simulink library "spacecraft_simulink_library"  (Simulink 7.8)
settings: Solver=ode45  SolverMode=SingleTasking  StartTime=0.0  StopTime=10.0  RelTol=1e-3
undefined symbols (not defined in the file or in its folder): I_sc, Krcs, q_bi0, sun_sensor_model_type, Trcs_saturation, w_bi0
settings Model: Creator=HARDAC_S  LastModifiedBy=HARDAC_S

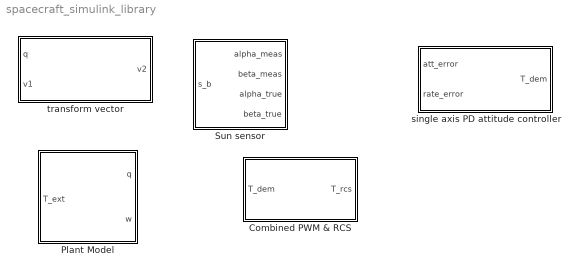
== system spacecraft_simulink_library ==
  Combined PWM & RCS : Subsystem  mask{T_deadband=[0 0 0], T_saturation=Trcs_saturation, K_rcs=[Krcs Krcs Krcs]}
      mask prompts: T_deadband "Torque deadbands [X Y Z] [Nm]"; T_saturation "Torque saturation [X Y Z] [Nm]"; K_rcs "RCS gain [X Y Z]"
  Plant Model : Subsystem
  Sun sensor : Subsystem
  single axis PD attitude controller : Subsystem  mask{Kp=0, Kd=0}
      mask prompts: Kp "Proportional gain Kp"; Kd "Derivative gain Kd"
  transform vector : MATLAB Function  TreatAsAtomicUnit=on

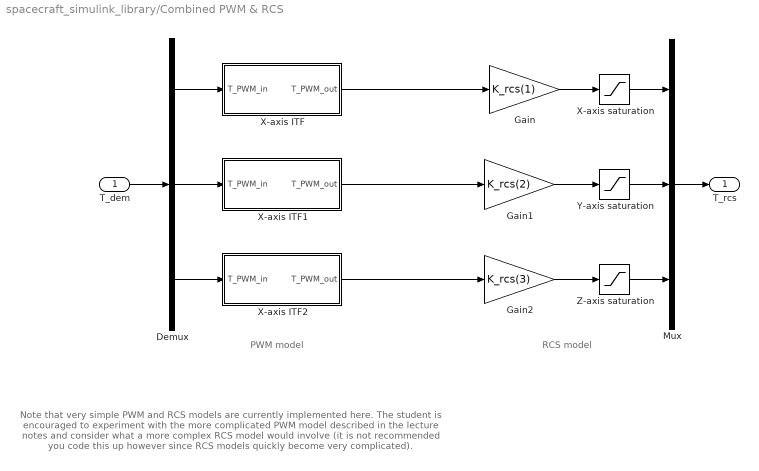
== system spacecraft_simulink_library/Combined PWM & RCS ==
  note: Note that very simple PWM and RCS models are currently implemented here. The student is
      | encouraged to experiment with the more complicated PWM model described in the lecture
      | notes and consider what a more complex RCS model would involve (it is not recommended
      | you code this up however since RCS models quickly become very complicated).
  note: RCS model
  note: PWM model
  T_dem : Inport
  Demux : Demux  Outputs=3
  Gain : Gain  Gain=K_rcs(1)  SaturateOnIntegerOverflow=on  OutDataTypeStr=Inherit: Same as input  ParamDataTypeStr=Inherit: Same as input
  Gain1 : Gain  Gain=K_rcs(2)  SaturateOnIntegerOverflow=on  OutDataTypeStr=Inherit: Same as input  ParamDataTypeStr=Inherit: Same as input
  Gain2 : Gain  Gain=K_rcs(3)  SaturateOnIntegerOverflow=on  OutDataTypeStr=Inherit: Same as input  ParamDataTypeStr=Inherit: Same as input
  Mux : Mux  Inputs=3
  X-axis ITF : Subsystem  mask{T_db=T_deadband(1)}
      mask prompts: T_db "Torque deadband [Nm]"
  X-axis ITF1 : Subsystem  mask{T_db=T_deadband(2)}
      mask prompts: T_db "Torque deadband [Nm]"
  X-axis ITF2 : Subsystem  mask{T_db=T_deadband(3)}
      mask prompts: T_db "Torque deadband [Nm]"
  X-axis saturation : Saturate  UpperLimit=+T_saturation(1)  LowerLimit=-T_saturation(1)
  Y-axis saturation : Saturate  UpperLimit=T_saturation(2)  LowerLimit=-T_saturation(2)
  Z-axis saturation : Saturate  UpperLimit=T_saturation(3)  LowerLimit=-T_saturation(3)
  T_rcs : Outport
  wires:
  Gain2/1 -> Z-axis saturation/1
  Gain1/1 -> Y-axis saturation/1
  Gain/1 -> X-axis saturation/1
  X-axis ITF2/1(T_PWM_out) -> Gain2/1
  X-axis ITF1/1(T_PWM_out) -> Gain1/1
  X-axis ITF/1(T_PWM_out) -> Gain/1
  T_dem/1 -> Demux/1
  Demux/3 -> X-axis ITF2/1(T_PWM_in)
  Demux/2 -> X-axis ITF1/1(T_PWM_in)
  Demux/1 -> X-axis ITF/1(T_PWM_in)
  Z-axis saturation/1 -> Mux/3
  Y-axis saturation/1 -> Mux/2
  X-axis saturation/1 -> Mux/1
  Mux/1 -> T_rcs/1

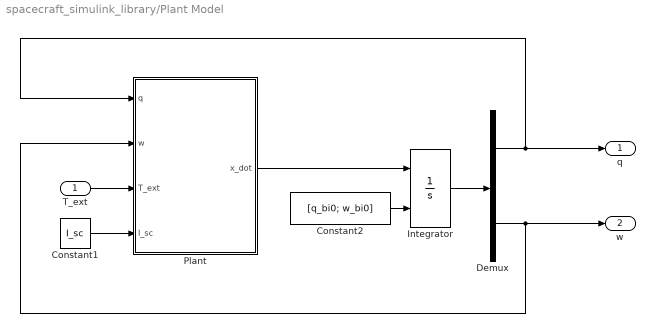
== system spacecraft_simulink_library/Plant Model ==
  T_ext : Inport
  Constant1 : Constant  Value=I_sc
  Constant2 : Constant  Value=[q_bi0; w_bi0]
  Demux : Demux  Outputs=[4 3]
  Integrator : Integrator  InitialConditionSource=external
  Plant : MATLAB Function  TreatAsAtomicUnit=on
  q : Outport
  w : Outport  Port=2
  wires:
  Plant/1(x_dot) -> Integrator/1
  Integrator/1 -> Demux/1
  Demux/1 -> q/1, Plant/1(q)
  Demux/2 -> w/1, Plant/2(w)
  T_ext/1 -> Plant/3(T_ext)
  Constant1/1 -> Plant/4(I_sc)
  Constant2/1 -> Integrator/2

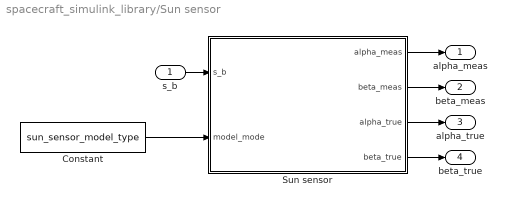
== system spacecraft_simulink_library/Sun sensor ==
  s_b : Inport
  Constant : Constant  Value=sun_sensor_model_type
  Sun sensor : MATLAB Function  TreatAsAtomicUnit=on
  alpha_meas : Outport
  beta_meas : Outport  Port=2
  alpha_true : Outport  Port=3
  beta_true : Outport  Port=4
  wires:
  Constant/1 -> Sun sensor/2(model_mode)
  s_b/1 -> Sun sensor/1(s_b)
  Sun sensor/1(alpha_meas) -> alpha_meas/1
  Sun sensor/2(beta_meas) -> beta_meas/1
  Sun sensor/3(alpha_true) -> alpha_true/1
  Sun sensor/4(beta_true) -> beta_true/1

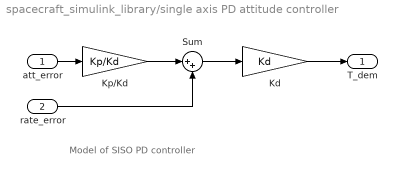
== system spacecraft_simulink_library/single axis PD attitude controller ==
  note: Model of SISO PD controller
  att_error : Inport
  rate_error : Inport  Port=2
  Kd : Gain  Gain=Kd  SaturateOnIntegerOverflow=on  OutDataTypeStr=Inherit: Same as input  ParamDataTypeStr=Inherit: Same as input
  Kp/Kd : Gain  Gain=Kp/Kd  SaturateOnIntegerOverflow=on  OutDataTypeStr=Inherit: Same as input  ParamDataTypeStr=Inherit: Same as input
  Sum : Sum  Inputs=|++  SaturateOnIntegerOverflow=on
  T_dem : Outport
  wires:
  Kp/Kd/1 -> Sum/1
  Sum/1 -> Kd/1
  Kd/1 -> T_dem/1
  att_error/1 -> Kp/Kd/1
  rate_error/1 -> Sum/2

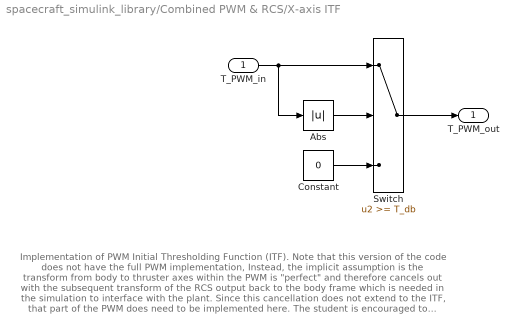
== system spacecraft_simulink_library/Combined PWM & RCS/X-axis ITF ==
  note: Implementation of PWM Initial Thresholding Function (ITF).
      |
      | Note that this version of the code does not have the full PWM implementation, Instead, the implicit assumption is the
      | transform from body to thruster axes within the PWM is "perfect" and therefore cancels out with the subsequent transform
      | of the RCS output back to the body frame which is needed in the simulation to interface with the plant. Since this
      | cancellation does not extend to the ITF, that part of the PWM does need to be implemented here.
      |
      | The student is encouraged to experiment with the "full" PWM described in the lecture notes to verify the above.
  T_PWM_in : Inport
  Abs : Abs  SaturateOnIntegerOverflow=on
  Constant : Constant  Value=0
  Switch : Switch  Threshold=T_db  SaturateOnIntegerOverflow=on
  T_PWM_out : Outport
  wires:
  Switch/1 -> T_PWM_out/1
  T_PWM_in/1 -> Abs/1, Switch/1
  Constant/1 -> Switch/3
  Abs/1 -> Switch/2

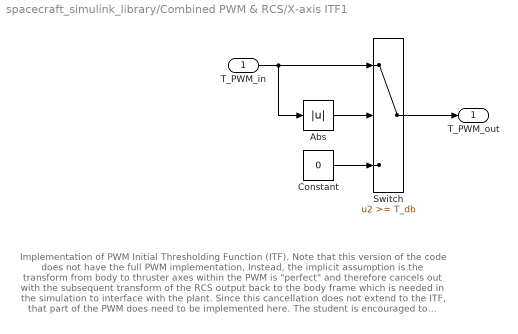
== system spacecraft_simulink_library/Combined PWM & RCS/X-axis ITF1 ==
  note: Implementation of PWM Initial Thresholding Function (ITF).
      |
      | Note that this version of the code does not have the full PWM implementation, Instead, the implicit assumption is the
      | transform from body to thruster axes within the PWM is "perfect" and therefore cancels out with the subsequent transform
      | of the RCS output back to the body frame which is needed in the simulation to interface with the plant. Since this
      | cancellation does not extend to the ITF, that part of the PWM does need to be implemented here.
      |
      | The student is encouraged to experiment with the "full" PWM described in the lecture notes to verify the above.
  T_PWM_in : Inport
  Abs : Abs  SaturateOnIntegerOverflow=on
  Constant : Constant  Value=0
  Switch : Switch  Threshold=T_db  SaturateOnIntegerOverflow=on
  T_PWM_out : Outport
  wires:
  Abs/1 -> Switch/2
  Constant/1 -> Switch/3
  T_PWM_in/1 -> Switch/1, Abs/1
  Switch/1 -> T_PWM_out/1

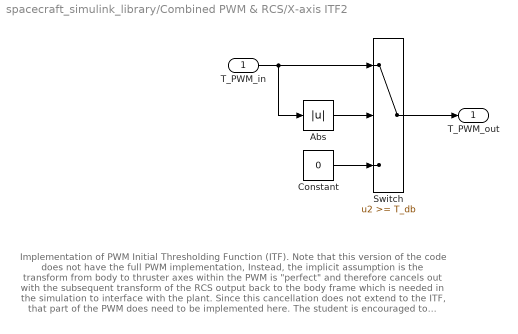
== system spacecraft_simulink_library/Combined PWM & RCS/X-axis ITF2 ==
  note: Implementation of PWM Initial Thresholding Function (ITF).
      |
      | Note that this version of the code does not have the full PWM implementation, Instead, the implicit assumption is the
      | transform from body to thruster axes within the PWM is "perfect" and therefore cancels out with the subsequent transform
      | of the RCS output back to the body frame which is needed in the simulation to interface with the plant. Since this
      | cancellation does not extend to the ITF, that part of the PWM does need to be implemented here.
      |
      | The student is encouraged to experiment with the "full" PWM described in the lecture notes to verify the above.
  T_PWM_in : Inport
  Abs : Abs  SaturateOnIntegerOverflow=on
  Constant : Constant  Value=0
  Switch : Switch  Threshold=T_db  SaturateOnIntegerOverflow=on
  T_PWM_out : Outport
  wires:
  Switch/1 -> T_PWM_out/1
  T_PWM_in/1 -> Abs/1, Switch/1
  Constant/1 -> Switch/3
  Abs/1 -> Switch/2

== matlab function Sun sensor/Sun sensor ==
  data: s_b input double; alpha_meas output double; model_mode input double; beta_meas output double; alpha_true output double; beta_true output double
function  [alpha_meas, beta_meas, alpha_true, beta_true] = SunSensor(s_b,model_mode)
% SunSensor. Models Sun sensor by converting input sun vector (in body
% frame) to Sun sensor [alpha, beta] angles.
%
% Format:
%   [alpha, beta] = SunSensor(s_b, model_mode)
% where:
%   u           is the sun vector in the body frame
%   model_mode  selects ideal sensor (=1) or non-linear sensor (=2)
%   angles      is [alpha, beta] angles measured by the sun sensor
% Uses the method described in section 4.1 of P6 notes

% calculate [alpha, beta] angles - note this algorithm only works when the
% sun vector lies within 90deg of the sensor boresight (=Z axis - see
% figure 3-8 of P4 notes)
alpha_true = atan2(+s_b(2),s_b(3));
beta_true  = atan2(-s_b(1),s_b(3));

% apply non-linear characteristic if requested by user input
if model_mode==2
    alpha_meas = SunSensorResponse(alpha_true);
    beta_meas  = SunSensorResponse(beta_true);
else
    alpha_meas = alpha_true;
    beta_meas  = beta_true;
end

return

% =========================================================================
% Private functions (can only be called from the SunSensor function
% =========================================================================
function meas_angle = SunSensorResponse(true_angle)
% SunSensorResponse. Implements the sun sensor response shown in lecture notes.
meas_angle     = 0;
true_angle_max = 83*pi/180;
meas_angle_max = 0.5*(sin(7*pi/180) + cos(7*pi/180)*tan(true_angle_max))./(1+tan(true_angle_max).^2).^0.5;
if abs(true_angle)<7*pi/180
	meas_angle = true_angle;
elseif true_angle>0&&true_angle<83*pi/180
    meas_angle = 0.5*(sin(7*pi/180) + cos(7*pi/180)*tan(true_angle))./(1+tan(true_angle).^2).^0.5;
elseif true_angle<0&&true_angle>-83*pi/180
    meas_angle = -0.5*(sin(7*pi/180) - cos(7*pi/180)*tan(true_angle))./(1+tan(true_angle).^2).^0.5;
elseif true_angle>=83*pi/180
    meas_angle = -meas_angle_max/(7*pi/180)*(true_angle-pi/2);
elseif true_angle<=-83*pi/180
    meas_angle = -meas_angle_max/(7*pi/180)*(true_angle+pi/2);
end

== matlab function Plant Model/Plant ==
  data: q input double; x_dot output double; w input double; T_ext input double; I_sc input double
function x_dot = fcn(q,w,T_ext,I_sc)

% derivative of quaternion part of state vector:
OMEGA   = [    0  w(3) -w(2)  w(1);
           -w(3)     0  w(1)  w(2);
            w(2) -w(1)     0  w(3);
           -w(1) -w(2) -w(3)     0];
q_dot   = 0.5*OMEGA*q;


% derivative of rate vector part of state vector:
w_dot   = inv(I_sc)*(T_ext - cross(w,I_sc*w));


% overall state vector derivative:
x_dot   = [q_dot; w_dot];

== matlab function transform vector ==
  data: q input double; v2 output double; v1 input double
function  v2 = TransformVector(q,v1)
% TransformVector. Transforms a vector from one frame to another. 
%
% Format:
%   v2 = TransformVector(q,v1)
% where:
%   q   is the quaternion representing the transformation
%   v1  is the vector being transformed.
%   v2  is the transformed vector.

% compute DCM
DCM = [q(1)^2-q(2)^2-q(3)^2+q(4)^2        2*(q(1)*q(2)+q(3)*q(4))        2*(q(1)*q(3)-q(2)*q(4));
           2*(q(1)*q(2)-q(3)*q(4))   -q(1)^2+q(2)^2-q(3)^2+q(4)^2	       2*(q(2)*q(3)+q(1)*q(4));
		   2*(q(1)*q(3)+q(2)*q(4))        2*(q(2)*q(3)-q(1)*q(4))   -q(1)^2-q(2)^2+q(3)^2+q(4)^2];
	   
% transform vector from one frame to another
v2  = DCM*v1;

return
